simulink model "Control_Arduino"  (R2023b)
settings: Solver=FixedStepDiscrete  StartTime=0.0  StopTime=90  FixedStep=0.01  RelTol=1e-3  EnableMultiTasking=on
undefined symbols (not defined in the file): L, R
libraries: simulink x36, arduinolib x17, canmsglib x4, arduinowifilib x2
settings Model: ExtModeTrigDuration=2  Creator=pablo  LastModifiedBy=pablo
settings SolverCC: AutoInsertRateTranBlk=on
settings OptimizationCC: EnhancedBackFolding=on  PassReuseOutputArgsAs=Individual arguments  ZeroExternalMemoryAtStartup=off  ZeroInternalMemoryAtStartup=off  MaxStackSize=64  OptimizeBlockOrder=speed  DifferentSizesBufferReuse=on  OptimizationCustomize=off  EfficientTunableParamExpr=on
settings DebuggingCC: ReadBeforeWriteMsg=DisableAll  WriteAfterWriteMsg=DisableAll  WriteAfterReadMsg=DisableAll  MultiTaskDSMMsg=none  ParameterTunabilityLossMsg=error
settings HardwareCC: ProdBitPerPointer=32  ProdBitPerSizeT=32  ProdBitPerPtrDiffT=32  ProdLargestAtomicInteger=Long  ProdLargestAtomicFloat=Double  ProdWordSize=32  ProdHWDeviceType=ARM Compatible->ARM Cortex
settings ModelReferenceCC: UpdateModelReferenceTargets=IfOutOfDate
settings SFSimCC: SFSimEcho=off  MATLABDynamicMemAlloc=off
settings RTWCC: Description=Embedded Coder  SystemTargetFile=ert.tlc  HardwareBoard=Arduino MKR WiFi 1010  TemplateMakefile=ert_default_tmf  Toolchain=Arduino ARM  BuildConfiguration=Faster Runs
settings CodeAppCC: ForceParamTrailComments=on  IgnoreCustomStorageClasses=off  OperatorAnnotations=on  SimulinkDataObjDesc=on  SFDataObjDesc=on  InsertBlockDesc=on
settings ERTTargetCC: SupportContinuousTime=on  SupportVariableSizeSignals=on  ExtModeTransport=3  ExtModeStaticAlloc=on  ExtModeAutomaticAllocSize=off  ExtModeStaticAllocSize=8192  ExtModeMexFile=ext_xcp  ExtModeIntrfLevel=Level2 - Open

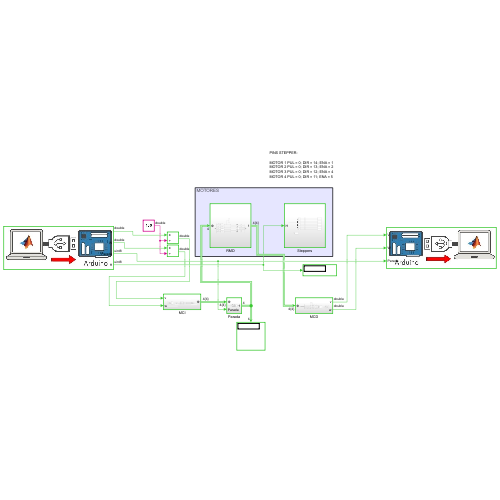
[thumbnail: Simulink's stored preview of the top-level diagram]
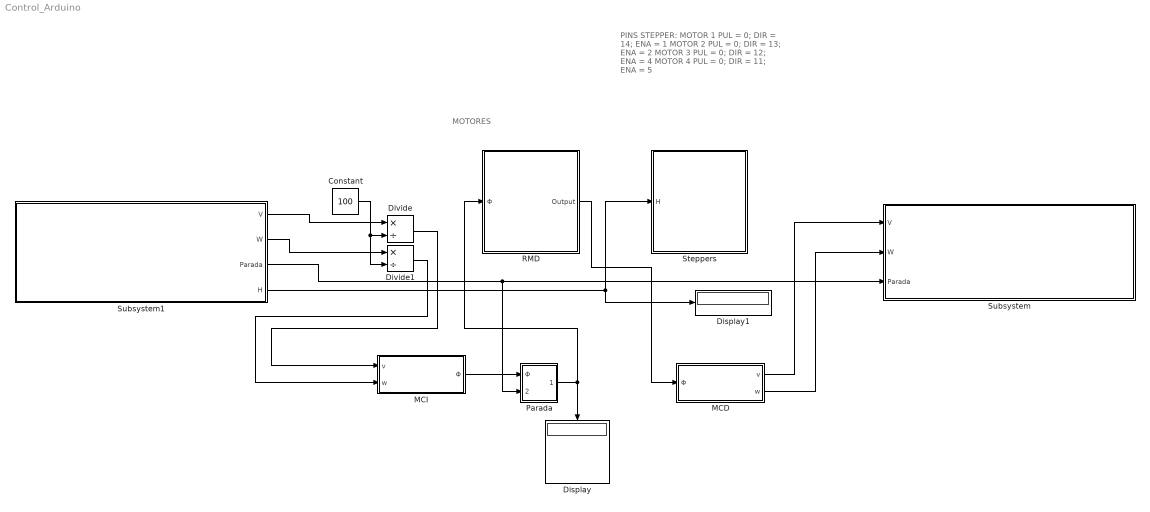
== system Control_Arduino ==
  note: PINS STEPPER:
      |
      | MOTOR 1 PUL = 0; DIR = 14; ENA = 1
      | MOTOR 2 PUL = 0; DIR = 13; ENA = 2
      | MOTOR 3 PUL = 0; DIR = 12; ENA = 4
      | MOTOR 4 PUL = 0; DIR = 11; ENA = 5
  note: MOTORES
  Constant : Constant  Value=100
  Display : Display
  Display1 : Display
      settings: Format=binary (Stored Integer)
  Divide : Product  Inputs=*/
  Divide1 : Product  Inputs=*/
  MCD : Subsystem
  MCI : Subsystem
  Parada : Subsystem
  RMD : Subsystem
  Steppers : Subsystem
  Subsystem : Subsystem
      mask Display: image('am.jpg');
  Subsystem1 : Subsystem
      mask Display: image('ma.jpg');
  wires:
  Subsystem1/1(V) -> Divide/1
  Subsystem1/2(W) -> Divide1/1
  Subsystem1/3(Parada) -> Subsystem/3(Parada), Parada/2(Parada)
  Constant/1 -> Divide1/2, Divide/2
  Divide/1 -> MCI/1(v)
  Divide1/1 -> MCI/2(w)
  MCD/1(v) -> Subsystem/1(V)
  MCD/2(w) -> Subsystem/2(W)
  MCI/1(Φ) -> Parada/1(Φ)
  Parada/1(Out1) -> RMD/1(Φ), Display/1
  RMD/1(Output) -> MCD/1(Φ)
  Subsystem1/4(H) -> Steppers/1(H), Display1/1

== system Control_Arduino/MCD ==
  Φ : Inport
  Bus Selector : BusSelector  OutputSignals=GPS1,GPS2,GPS3,GPS4
  Constant : Constant  Value=2
  Demux : Demux  Outputs=2
  Divide2 : Product  Inputs=*/
  Divide3 : Product  Inputs=*/
  Gain1 : Gain  Gain=[1/2 1/2; -1/L 1/L]  Multiplication=Matrix(K*u) (u vector)
  Gain2 : Gain  Gain=R
  Gain3 : Gain  Gain=R
  Mux : Mux  Inputs=2
  Sum : Sum  Inputs=|++
  Sum1 : Sum  Inputs=|++
  v : Outport
  w : Outport  Port=2
  wires:
  Sum1/1 -> Divide2/1
  Φ/1 -> Bus Selector/1
  Constant/1 -> Divide3/2, Divide2/2
  Sum/1 -> Divide3/1
  Gain2/1 -> Mux/1
  Gain3/1 -> Mux/2
  Mux/1 -> Gain1/1
  Gain1/1 -> Demux/1
  Demux/1 -> v/1
  Demux/2 -> w/1
  Divide2/1 -> Gain2/1
  Divide3/1 -> Gain3/1
  Bus Selector/1 -> Sum1/1  "<GPS1>"
  Bus Selector/2 -> Sum1/2  "<GPS2>"
  Bus Selector/3 -> Sum/1  "<GPS3>"
  Bus Selector/4 -> Sum/2  "<GPS4>"

== system Control_Arduino/MCI ==
  note: velocidad en grados por segundo
  note: L = distancia entre el eje de las ruedas izquierda y derecha
  note: radio de las ruedas
  note: Velocidades angulares:
      | 1. Frente izquierda
      | 2. Trasera izquierda
      | 3. Frente derecha
      | 4. Trasera derecha
  v : Inport
  w : Inport  Port=2
  Bus Creator : BusCreator  Inputs=4
  Demux : Demux  Outputs=2
  Gain : Gain  Gain=[1 -L/2; 1 L/2]  Multiplication=Matrix(K*u) (u vector)
  Gain1 : Gain  Gain=10
  Gain2 : Gain  Gain=1/R
  Gain3 : Gain  Gain=10
  Mux : Mux  Inputs=2
  Rate Limiter : RateLimiter  RisingSlewLimit=9  FallingSlewLimit=-9  SampleTimeMode=inherited
  Rate Limiter1 : RateLimiter  RisingSlewLimit=9  FallingSlewLimit=-9  SampleTimeMode=inherited
  Φ : Outport
  wires:
  Bus Creator/1 -> Φ/1
  Mux/1 -> Gain/1
  v/1 -> Mux/1
  w/1 -> Mux/2
  Demux/1 -> Rate Limiter/1
  Demux/2 -> Rate Limiter1/1
  Gain/1 -> Gain2/1
  Gain2/1 -> Demux/1
  Gain1/1 -> Bus Creator/2, Bus Creator/1
  Rate Limiter1/1 -> Gain3/1
  Rate Limiter/1 -> Gain1/1
  Gain3/1 -> Bus Creator/4, Bus Creator/3

== system Control_Arduino/Parada ==
  Φ : Inport
  Parada : Inport  Port=2
  Bus Creator : BusCreator  Inputs=4
  Constant : Constant  Value=0
  Switch : Switch  Criteria=u2 ~= 0  SaturateOnIntegerOverflow=off  InputSameDT=off
  Out1 : Outport
  wires:
  Switch/1 -> Out1/1
  Φ/1 -> Switch/3
  Parada/1 -> Switch/2
  Bus Creator/1 -> Switch/1
  Constant/1 -> Bus Creator/2, Bus Creator/4, Bus Creator/3, Bus Creator/1

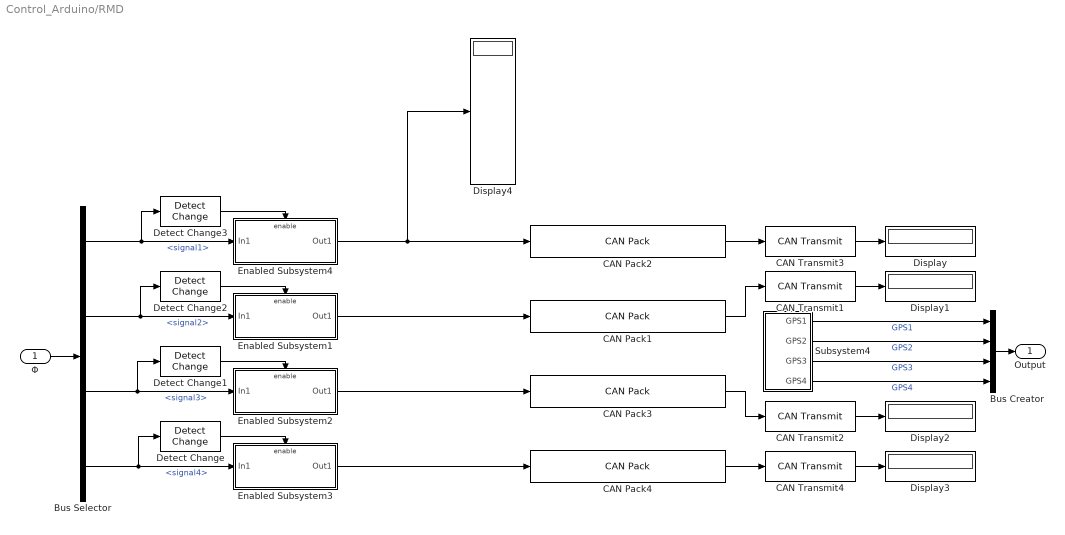
== system Control_Arduino/RMD ==
  Φ : Inport
  Bus Creator : BusCreator  Inputs=4
  Bus Selector : BusSelector  OutputSignals=signal1,signal2,signal3,signal4
  CAN Pack1 : canmsglib/CAN Pack  MsgList=(none)  MsgName=CAN Msg  MsgIDType=Standard (11-bit identifier)  MsgIdentifier=322  MsgLength=8  Remote=off  ApplyMinMax=off  BusOutput=on  SignalInfo={ 'position', '8', '16', 'BE', 'signed', 'Standard', '0', '1', '-95.5', '-95.5', '95.5'; 'velocity', '28', '12', 'BE', 'signed', 'Standard', '0', '1', '-45', '-45', '45'; 'kp', '32', '12', 'BE', 'unsigned', 'Standard', '0', '1', '0', '0', '500'; 'kd', '52', '12', 'BE', 'unsigned', 'Standard', '0', '1', '0', '0', '5'; 'torque', '56', '12', 'BE', 'signed', 'Standard', '0', '1', '-18', '-18', '18' }
      settings: LibrarySourceBlock=embeddedtargetslib/Host Communication/CAN Pack  DataFormat=raw data
  CAN Pack2 : canmsglib/CAN Pack  MsgList=(none)  MsgName=CAN Msg  MsgIDType=Standard (11-bit identifier)  MsgIdentifier=321  MsgLength=8  Remote=off  ApplyMinMax=off  BusOutput=on  SignalInfo={ 'position', '8', '16', 'BE', 'signed', 'Standard', '0', '1', '-95.5', '-95.5', '95.5'; 'velocity', '28', '12', 'BE', 'signed', 'Standard', '0', '1', '-45', '-45', '45'; 'kp', '32', '12', 'BE', 'unsigned', 'Standard', '0', '1', '0', '0', '500'; 'kd', '52', '12', 'BE', 'unsigned', 'Standard', '0', '1', '0', '0', '5'; 'torque', '56', '12', 'BE', 'signed', 'Standard', '0', '1', '-18', '-18', '18' }
      settings: LibrarySourceBlock=embeddedtargetslib/Host Communication/CAN Pack  DataFormat=raw data
  CAN Pack3 : canmsglib/CAN Pack  MsgList=(none)  MsgName=CAN Msg  MsgIDType=Standard (11-bit identifier)  MsgIdentifier=323  MsgLength=8  Remote=off  ApplyMinMax=off  BusOutput=on  SignalInfo={ 'position', '8', '16', 'BE', 'signed', 'Standard', '0', '1', '-95.5', '-95.5', '95.5'; 'velocity', '28', '12', 'BE', 'signed', 'Standard', '0', '1', '-45', '-45', '45'; 'kp', '32', '12', 'BE', 'unsigned', 'Standard', '0', '1', '0', '0', '500'; 'kd', '52', '12', 'BE', 'unsigned', 'Standard', '0', '1', '0', '0', '5'; 'torque', '56', '12', 'BE', 'signed', 'Standard', '0', '1', '-18', '-18', '18' }
      settings: LibrarySourceBlock=embeddedtargetslib/Host Communication/CAN Pack  DataFormat=raw data
  CAN Pack4 : canmsglib/CAN Pack  MsgList=(none)  MsgName=CAN Msg  MsgIDType=Standard (11-bit identifier)  MsgIdentifier=324  MsgLength=8  Remote=off  ApplyMinMax=off  BusOutput=on  SignalInfo={ 'position', '8', '16', 'BE', 'signed', 'Standard', '0', '1', '-95.5', '-95.5', '95.5'; 'velocity', '28', '12', 'BE', 'signed', 'Standard', '0', '1', '-45', '-45', '45'; 'kp', '32', '12', 'BE', 'unsigned', 'Standard', '0', '1', '0', '0', '500'; 'kd', '52', '12', 'BE', 'unsigned', 'Standard', '0', '1', '0', '0', '5'; 'torque', '56', '12', 'BE', 'signed', 'Standard', '0', '1', '-18', '-18', '18' }
      settings: LibrarySourceBlock=embeddedtargetslib/Host Communication/CAN Pack  DataFormat=raw data
  CAN Transmit{1..4} (4 alike) : arduinolib/CAN Transmit  inputDataType=CAN Msg  BlockingMode_=on  BlockTimeout_=1  outputStatus=on  identifierType=Standard (11-bit identifier)  messageId=100  msgLength=8  remoteFrame=off
  Detect Change{,1..3} (4 alike) : simulink/Logic and Bit Operations/Detect Change  vinit=0  OutDataTypeStr=boolean
  Display{,1..4} (5 alike) : Display
      Display settings: Format=binary (Stored Integer)
      Display1 settings: Format=binary (Stored Integer)
      Display2 settings: Format=binary (Stored Integer)
      Display3 settings: Format=binary (Stored Integer)
      Display4 settings: Format=hex (Stored Integer)
  Enabled Subsystem1 : Subsystem  TreatAsAtomicUnit=on
  Enabled Subsystem2 : Subsystem  TreatAsAtomicUnit=on
  Enabled Subsystem3 : Subsystem  TreatAsAtomicUnit=on
  Enabled Subsystem4 : Subsystem  TreatAsAtomicUnit=on
  Subsystem4 : Subsystem
  Output : Outport
  wires:
  Enabled Subsystem4/1(Out1) -> Display4/1, CAN Pack2/1
  Enabled Subsystem1/1(Out1) -> CAN Pack1/1
  Enabled Subsystem2/1(Out1) -> CAN Pack3/1
  Enabled Subsystem3/1(Out1) -> CAN Pack4/1
  CAN Pack2/1 -> CAN Transmit3/1
  CAN Pack4/1 -> CAN Transmit4/1
  CAN Transmit3/1 -> Display/1
  CAN Transmit1/1 -> Display1/1
  CAN Transmit2/1 -> Display2/1
  CAN Transmit4/1 -> Display3/1
  CAN Pack1/1 -> CAN Transmit1/1
  CAN Pack3/1 -> CAN Transmit2/1
  Detect Change/1 -> Enabled Subsystem3/Enable
  Detect Change1/1 -> Enabled Subsystem2/Enable
  Detect Change2/1 -> Enabled Subsystem1/Enable
  Detect Change3/1 -> Enabled Subsystem4/Enable
  Φ/1 -> Bus Selector/1
  Bus Selector/1 -> Enabled Subsystem4/1(In1), Detect Change3/1  "<signal1>"
  Bus Selector/2 -> Detect Change2/1, Enabled Subsystem1/1(In1)  "<signal2>"
  Bus Selector/3 -> Detect Change1/1, Enabled Subsystem2/1(In1)  "<signal3>"
  Bus Selector/4 -> Detect Change/1, Enabled Subsystem3/1(In1)  "<signal4>"
  Subsystem4/1(GPS1) -> Bus Creator/1  "GPS1"
  Subsystem4/2(GPS2) -> Bus Creator/2  "GPS2"
  Subsystem4/3(GPS3) -> Bus Creator/3  "GPS3"
  Subsystem4/4(GPS4) -> Bus Creator/4  "GPS4"
  Bus Creator/1 -> Output/1

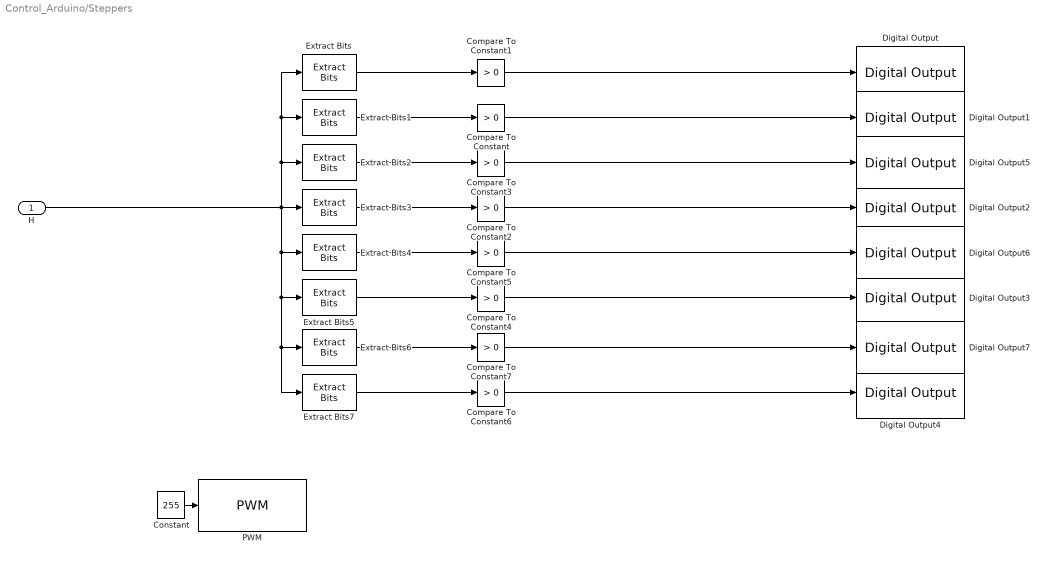
== system Control_Arduino/Steppers ==
  H : Inport
  Compare To Constant{,1..7} (8 alike) : simulink/Logic and Bit Operations/Compare To Constant  relop=>  const=0  OutDataTypeStr=uint8
  Constant : Constant  Value=255
  Digital Output : arduinolib/Digital Output  pinNumber=1  Direction=output  blockPlatform=arduino
  Digital Output1 : arduinolib/Digital Output  pinNumber=14  Direction=output  blockPlatform=arduino
  Digital Output2 : arduinolib/Digital Output  pinNumber=13  Direction=output  blockPlatform=arduino
  Digital Output3 : arduinolib/Digital Output  pinNumber=12  Direction=output  blockPlatform=arduino
  Digital Output4 : arduinolib/Digital Output  pinNumber=11  Direction=output  blockPlatform=arduino
  Digital Output5 : arduinolib/Digital Output  pinNumber=2  Direction=output  blockPlatform=arduino
  Digital Output6 : arduinolib/Digital Output  pinNumber=4  Direction=output  blockPlatform=arduino
  Digital Output7 : arduinolib/Digital Output  pinNumber=5  Direction=output  blockPlatform=arduino
  Extract Bits : simulink/Logic and Bit Operations/Extract Bits  bitsToExtract=Range of bits  numBits=8  bitIdxRange=4  outScalingMode=Preserve fixed-point scaling
  Extract Bits1 : simulink/Logic and Bit Operations/Extract Bits  bitsToExtract=Range of bits  numBits=8  bitIdxRange=0  outScalingMode=Preserve fixed-point scaling
  Extract Bits2 : simulink/Logic and Bit Operations/Extract Bits  bitsToExtract=Range of bits  numBits=8  bitIdxRange=5  outScalingMode=Preserve fixed-point scaling
  Extract Bits3 : simulink/Logic and Bit Operations/Extract Bits  bitsToExtract=Range of bits  numBits=8  bitIdxRange=1  outScalingMode=Preserve fixed-point scaling
  Extract Bits4 : simulink/Logic and Bit Operations/Extract Bits  bitsToExtract=Range of bits  numBits=8  bitIdxRange=6  outScalingMode=Preserve fixed-point scaling
  Extract Bits5 : simulink/Logic and Bit Operations/Extract Bits  bitsToExtract=Range of bits  numBits=8  bitIdxRange=2  outScalingMode=Preserve fixed-point scaling
  Extract Bits6 : simulink/Logic and Bit Operations/Extract Bits  bitsToExtract=Range of bits  numBits=8  bitIdxRange=7  outScalingMode=Preserve fixed-point scaling
  Extract Bits7 : simulink/Logic and Bit Operations/Extract Bits  bitsToExtract=Range of bits  numBits=8  bitIdxRange=3  outScalingMode=Preserve fixed-point scaling
  PWM : arduinolib/PWM  pinNumber=0  frequencyType=Default  desiredFrequency=490.2  achievableFrequency=490.2
  wires:
  Extract Bits5/1 -> Compare To Constant4/1
  Compare To Constant3/1 -> Digital Output5/1
  Compare To Constant5/1 -> Digital Output6/1
  Compare To Constant2/1 -> Digital Output2/1
  Extract Bits7/1 -> Compare To Constant6/1
  Compare To Constant4/1 -> Digital Output3/1
  Compare To Constant7/1 -> Digital Output7/1
  Extract Bits/1 -> Compare To Constant1/1
  Compare To Constant/1 -> Digital Output1/1
  Compare To Constant1/1 -> Digital Output/1
  Extract Bits2/1 -> Compare To Constant3/1
  Extract Bits4/1 -> Compare To Constant5/1
  Compare To Constant6/1 -> Digital Output4/1
  Extract Bits3/1 -> Compare To Constant2/1
  Extract Bits1/1 -> Compare To Constant/1
  Extract Bits6/1 -> Compare To Constant7/1
  H/1 -> Extract Bits3/1, Extract Bits2/1, Extract Bits1/1, Extract Bits/1, Extract Bits4/1, Extract Bits5/1, Extract Bits7/1, Extract Bits6/1
  Constant/1 -> PWM/1

== system Control_Arduino/Subsystem ==
  V : Inport
  W : Inport  Port=2
  Parada : Inport  Port=3
  Data Type Conversion1 : DataTypeConversion  OutDataTypeStr=int16  ConvertRealWorld=Stored Integer (SI)  SaturateOnIntegerOverflow=off  RndMeth=Floor
  Data Type Conversion6 : DataTypeConversion  OutDataTypeStr=int16  ConvertRealWorld=Stored Integer (SI)  SaturateOnIntegerOverflow=off  RndMeth=Floor
  Data Type Conversion7 : DataTypeConversion  OutDataTypeStr=int16  ConvertRealWorld=Stored Integer (SI)  SaturateOnIntegerOverflow=off  RndMeth=Floor
  Display : Display
  Gain : Gain  Gain=100
  Gain5 : Gain  Gain=100
  Mux : Mux  Inputs=3
  WiFi UDP Send : arduinowifilib/WiFi UDP Send  remoteIPOctetString=192.168.137.1  remoteport=8888  localport=9090  remoteipoctet1=192  remoteipoctet2=168  remoteipoctet3=137  remoteipoctet4=1  wifiUDPIndex=0  blockPlatform=ARDUINO  isARMArch=true
  wires:
  Mux/1 -> Display/1, WiFi UDP Send/1
  V/1 -> Gain/1
  W/1 -> Gain5/1
  Data Type Conversion6/1 -> Mux/2
  Data Type Conversion7/1 -> Mux/3
  Gain/1 -> Data Type Conversion1/1
  Gain5/1 -> Data Type Conversion6/1
  Parada/1 -> Data Type Conversion7/1
  Data Type Conversion1/1 -> Mux/1

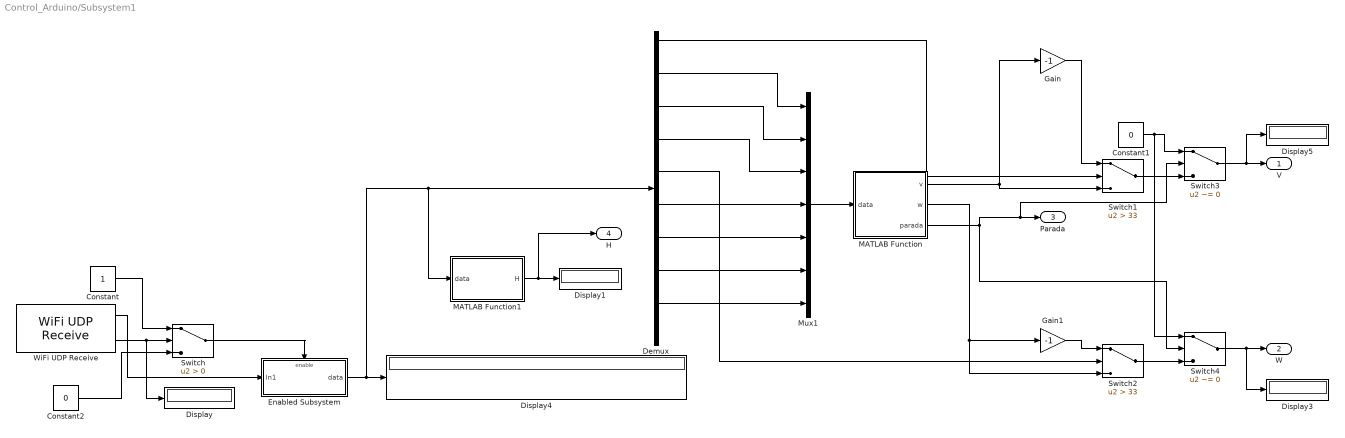
== system Control_Arduino/Subsystem1 ==
  Constant : Constant  OutDataTypeStr=boolean
  Constant1 : Constant  Value=0
  Constant2 : Constant  Value=0  OutDataTypeStr=boolean
  Demux : Demux  Outputs=10
  Display{,1,3..5} (5 alike) : Display
      Display1 settings: Format=binary (Stored Integer)
  Enabled Subsystem : Subsystem  TreatAsAtomicUnit=on
  Gain : Gain  Gain=-1
  Gain1 : Gain  Gain=-1
  MATLAB Function : MATLAB Function  TreatAsAtomicUnit=on
  MATLAB Function1 : MATLAB Function  TreatAsAtomicUnit=on
  Mux1 : Mux  Inputs=7
  Switch : Switch  Criteria=u2 > Threshold  SaturateOnIntegerOverflow=off  InputSameDT=off
  Switch1 : Switch  Criteria=u2 > Threshold  Threshold=33  SaturateOnIntegerOverflow=off  InputSameDT=off
  Switch2 : Switch  Criteria=u2 > Threshold  Threshold=33  SaturateOnIntegerOverflow=off  InputSameDT=off
  Switch3 : Switch  Criteria=u2 ~= 0  SaturateOnIntegerOverflow=off  InputSameDT=off
  Switch4 : Switch  Criteria=u2 ~= 0  SaturateOnIntegerOverflow=off  InputSameDT=off
  WiFi UDP Receive : arduinowifilib/WiFi UDP Receive  localport=9090  DataType=uint8  DataLength=10  SampleTime_=0.1  wifiUDPIndex=0  blockPlatform=ARDUINO  isARMArch=true
  V : Outport
  W : Outport  Port=2
  Parada : Outport  Port=3
  H : Outport  Port=4
  wires:
  Enabled Subsystem/1(data) -> Display4/1, Demux/1, MATLAB Function1/1(data)
  Constant/1 -> Switch/1
  WiFi UDP Receive/1 -> Enabled Subsystem/1(In1)
  Demux/1 -> Switch1/2
  Demux/2 -> Mux1/1
  WiFi UDP Receive/2 -> Switch/2, Display/1
  Demux/4 -> Mux1/3
  Demux/3 -> Mux1/2
  Switch/1 -> Enabled Subsystem/Enable
  Demux/6 -> Mux1/4
  Demux/5 -> Switch2/2
  Demux/8 -> Mux1/6
  Demux/7 -> Mux1/5
  Demux/9 -> Mux1/7
  Mux1/1 -> MATLAB Function/1(data)
  MATLAB Function/1(v) -> Switch1/3, Gain/1
  MATLAB Function/2(w) -> Switch2/3, Gain1/1
  MATLAB Function/3(parada) -> Switch4/2, Switch3/2, Parada/1
  Gain/1 -> Switch1/1
  Gain1/1 -> Switch2/1
  Constant1/1 -> Switch4/1, Switch3/1
  Switch2/1 -> Switch4/3
  Switch1/1 -> Switch3/3
  Switch4/1 -> W/1, Display3/1
  Switch3/1 -> V/1, Display5/1
  MATLAB Function1/1(H) -> H/1, Display1/1
  Constant2/1 -> Switch/3

== system Control_Arduino/RMD/Enabled Subsystem1 ==
  In1 : Inport
  Enable : EnablePort
  Gain : Gain  Gain=100
  Subsystem : Subsystem
  Out1 : Outport
  wires:
  In1/1 -> Gain/1
  Subsystem/1(Out1) -> Out1/1
  Gain/1 -> Subsystem/1(In1)

== system Control_Arduino/RMD/Enabled Subsystem2 ==
  In1 : Inport
  Enable : EnablePort
  Gain : Gain  Gain=100
  Subsystem : Subsystem
  Out1 : Outport
  wires:
  In1/1 -> Gain/1
  Subsystem/1(Out1) -> Out1/1
  Gain/1 -> Subsystem/1(In1)

== system Control_Arduino/RMD/Enabled Subsystem3 ==
  In1 : Inport
  Enable : EnablePort
  Gain : Gain  Gain=100
  Subsystem : Subsystem
  Out1 : Outport
  wires:
  In1/1 -> Gain/1
  Subsystem/1(Out1) -> Out1/1
  Gain/1 -> Subsystem/1(In1)

== system Control_Arduino/RMD/Enabled Subsystem4 ==
  In1 : Inport
  Enable : EnablePort
  Gain : Gain  Gain=100
  Subsystem : Subsystem
  Out1 : Outport
  wires:
  In1/1 -> Gain/1
  Subsystem/1(Out1) -> Out1/1
  Gain/1 -> Subsystem/1(In1)

== system Control_Arduino/RMD/Subsystem4 ==
  CAN Receive : arduinolib/CAN Receive  outputDataType=Raw data  identifierType=Standard (11-bit identifier)  messageId=577  msgLength=8  SampleTime=0.1  outputError=off  outputRemote=off
  CAN Receive1 : arduinolib/CAN Receive  outputDataType=Raw data  identifierType=Standard (11-bit identifier)  messageId=578  msgLength=8  SampleTime=0.1  outputError=off  outputRemote=off
  CAN Receive2 : arduinolib/CAN Receive  outputDataType=Raw data  identifierType=Standard (11-bit identifier)  messageId=579  msgLength=8  SampleTime=0.1  outputError=off  outputRemote=off
  CAN Receive3 : arduinolib/CAN Receive  outputDataType=Raw data  identifierType=Standard (11-bit identifier)  messageId=580  msgLength=8  SampleTime=0.1  outputError=off  outputRemote=off
  Subsystem : Subsystem
  Subsystem1 : Subsystem
  Subsystem2 : Subsystem
  Subsystem3 : Subsystem
  GPS1 : Outport
  GPS2 : Outport  Port=2
  GPS3 : Outport  Port=3
  GPS4 : Outport  Port=4
  wires:
  CAN Receive1/1 -> Subsystem2/1(In1)
  CAN Receive3/1 -> Subsystem/1(In1)
  CAN Receive2/1 -> Subsystem3/1(In1)
  CAN Receive/1 -> Subsystem1/1(In1)
  CAN Receive1/2 -> Subsystem2/Enable
  CAN Receive3/2 -> Subsystem/Enable
  CAN Receive2/2 -> Subsystem3/Enable
  CAN Receive/2 -> Subsystem1/Enable
  Subsystem1/1(GPS1) -> GPS1/1
  Subsystem3/1(GPS3) -> GPS3/1
  Subsystem/1(GPS4) -> GPS4/1
  Subsystem2/1(GPS2) -> GPS2/1

== system Control_Arduino/Subsystem1/Enabled Subsystem ==
  In1 : Inport
  Enable : EnablePort
  data : Outport
  wires:
  In1/1 -> data/1

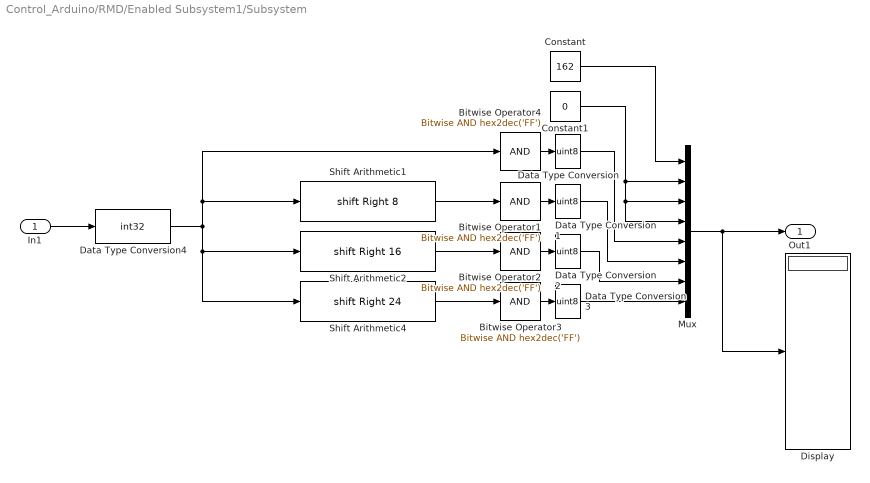
== system Control_Arduino/RMD/Enabled Subsystem1/Subsystem ==
  In1 : Inport
  Bitwise Operator{1..4} (4 alike) : simulink/Logic and Bit Operations/Bitwise Operator  logicop=AND  UseBitMask=on  BitMask=hex2dec('FF')  BitMaskRealWorld=Stored Integer
  Constant : Constant  Value=162  OutDataTypeStr=uint8
  Constant1 : Constant  Value=0  OutDataTypeStr=uint8
  Data Type Conversion{,1..3} (4 alike) : DataTypeConversion  OutDataTypeStr=uint8  ConvertRealWorld=Stored Integer (SI)  SaturateOnIntegerOverflow=off  RndMeth=Floor
  Data Type Conversion4 : DataTypeConversion  OutDataTypeStr=int32  SaturateOnIntegerOverflow=off  RndMeth=Floor
  Display : Display
  Mux : Mux  Inputs=8
  Shift Arithmetic1 : ArithShift  BitShiftNumber=8  BinPtShiftNumber=32  BitShiftDirection=Right
  Shift Arithmetic2 : ArithShift  BitShiftNumber=16  BinPtShiftNumber=32  BitShiftDirection=Right
  Shift Arithmetic4 : ArithShift  BitShiftNumber=24  BinPtShiftNumber=32  BitShiftDirection=Right
  Out1 : Outport
  wires:
  Bitwise Operator4/1 -> Data Type Conversion/1
  Shift Arithmetic1/1 -> Bitwise Operator1/1
  Bitwise Operator1/1 -> Data Type Conversion1/1
  Shift Arithmetic2/1 -> Bitwise Operator2/1
  Bitwise Operator2/1 -> Data Type Conversion2/1
  Shift Arithmetic4/1 -> Bitwise Operator3/1
  Bitwise Operator3/1 -> Data Type Conversion3/1
  Data Type Conversion4/1 -> Shift Arithmetic2/1, Shift Arithmetic4/1, Shift Arithmetic1/1, Bitwise Operator4/1
  In1/1 -> Data Type Conversion4/1
  Mux/1 -> Display/1, Out1/1
  Constant/1 -> Mux/1
  Constant1/1 -> Mux/4, Mux/3, Mux/2
  Data Type Conversion/1 -> Mux/5
  Data Type Conversion1/1 -> Mux/6
  Data Type Conversion2/1 -> Mux/7
  Data Type Conversion3/1 -> Mux/8

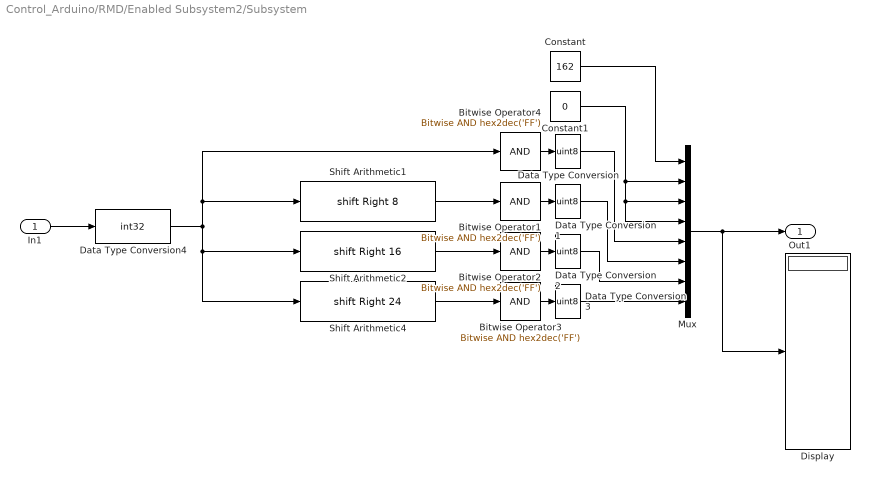
== system Control_Arduino/RMD/Enabled Subsystem2/Subsystem ==
  In1 : Inport
  Bitwise Operator{1..4} (4 alike) : simulink/Logic and Bit Operations/Bitwise Operator  logicop=AND  UseBitMask=on  BitMask=hex2dec('FF')  BitMaskRealWorld=Stored Integer
  Constant : Constant  Value=162  OutDataTypeStr=uint8
  Constant1 : Constant  Value=0  OutDataTypeStr=uint8
  Data Type Conversion{,1..3} (4 alike) : DataTypeConversion  OutDataTypeStr=uint8  ConvertRealWorld=Stored Integer (SI)  SaturateOnIntegerOverflow=off  RndMeth=Floor
  Data Type Conversion4 : DataTypeConversion  OutDataTypeStr=int32  SaturateOnIntegerOverflow=off  RndMeth=Floor
  Display : Display
  Mux : Mux  Inputs=8
  Shift Arithmetic1 : ArithShift  BitShiftNumber=8  BinPtShiftNumber=32  BitShiftDirection=Right
  Shift Arithmetic2 : ArithShift  BitShiftNumber=16  BinPtShiftNumber=32  BitShiftDirection=Right
  Shift Arithmetic4 : ArithShift  BitShiftNumber=24  BinPtShiftNumber=32  BitShiftDirection=Right
  Out1 : Outport
  wires:
  Bitwise Operator4/1 -> Data Type Conversion/1
  Shift Arithmetic1/1 -> Bitwise Operator1/1
  Bitwise Operator1/1 -> Data Type Conversion1/1
  Shift Arithmetic2/1 -> Bitwise Operator2/1
  Bitwise Operator2/1 -> Data Type Conversion2/1
  Shift Arithmetic4/1 -> Bitwise Operator3/1
  Bitwise Operator3/1 -> Data Type Conversion3/1
  Data Type Conversion4/1 -> Shift Arithmetic2/1, Shift Arithmetic4/1, Shift Arithmetic1/1, Bitwise Operator4/1
  In1/1 -> Data Type Conversion4/1
  Mux/1 -> Display/1, Out1/1
  Constant/1 -> Mux/1
  Constant1/1 -> Mux/4, Mux/3, Mux/2
  Data Type Conversion/1 -> Mux/5
  Data Type Conversion1/1 -> Mux/6
  Data Type Conversion2/1 -> Mux/7
  Data Type Conversion3/1 -> Mux/8

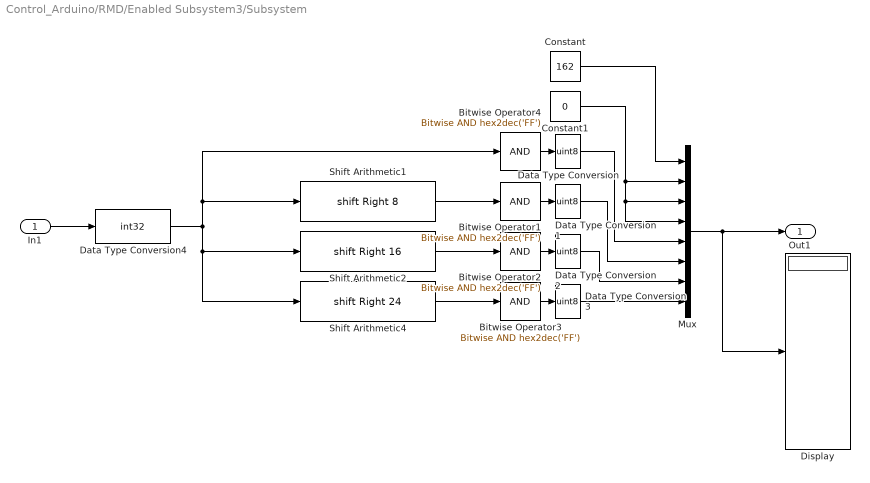
== system Control_Arduino/RMD/Enabled Subsystem3/Subsystem ==
  In1 : Inport
  Bitwise Operator{1..4} (4 alike) : simulink/Logic and Bit Operations/Bitwise Operator  logicop=AND  UseBitMask=on  BitMask=hex2dec('FF')  BitMaskRealWorld=Stored Integer
  Constant : Constant  Value=162  OutDataTypeStr=uint8
  Constant1 : Constant  Value=0  OutDataTypeStr=uint8
  Data Type Conversion{,1..3} (4 alike) : DataTypeConversion  OutDataTypeStr=uint8  ConvertRealWorld=Stored Integer (SI)  SaturateOnIntegerOverflow=off  RndMeth=Floor
  Data Type Conversion4 : DataTypeConversion  OutDataTypeStr=int32  SaturateOnIntegerOverflow=off  RndMeth=Floor
  Display : Display
  Mux : Mux  Inputs=8
  Shift Arithmetic1 : ArithShift  BitShiftNumber=8  BinPtShiftNumber=32  BitShiftDirection=Right
  Shift Arithmetic2 : ArithShift  BitShiftNumber=16  BinPtShiftNumber=32  BitShiftDirection=Right
  Shift Arithmetic4 : ArithShift  BitShiftNumber=24  BinPtShiftNumber=32  BitShiftDirection=Right
  Out1 : Outport
  wires:
  Bitwise Operator4/1 -> Data Type Conversion/1
  Shift Arithmetic1/1 -> Bitwise Operator1/1
  Bitwise Operator1/1 -> Data Type Conversion1/1
  Shift Arithmetic2/1 -> Bitwise Operator2/1
  Bitwise Operator2/1 -> Data Type Conversion2/1
  Shift Arithmetic4/1 -> Bitwise Operator3/1
  Bitwise Operator3/1 -> Data Type Conversion3/1
  Data Type Conversion4/1 -> Shift Arithmetic2/1, Shift Arithmetic4/1, Shift Arithmetic1/1, Bitwise Operator4/1
  In1/1 -> Data Type Conversion4/1
  Mux/1 -> Display/1, Out1/1
  Constant/1 -> Mux/1
  Constant1/1 -> Mux/4, Mux/3, Mux/2
  Data Type Conversion/1 -> Mux/5
  Data Type Conversion1/1 -> Mux/6
  Data Type Conversion2/1 -> Mux/7
  Data Type Conversion3/1 -> Mux/8

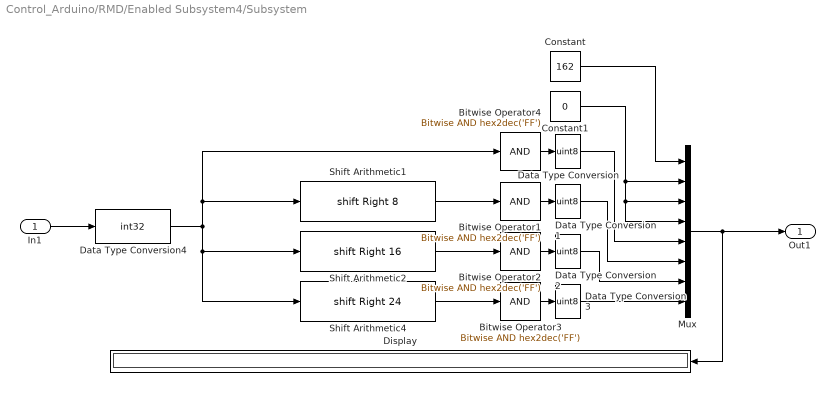
== system Control_Arduino/RMD/Enabled Subsystem4/Subsystem ==
  In1 : Inport
  Bitwise Operator{1..4} (4 alike) : simulink/Logic and Bit Operations/Bitwise Operator  logicop=AND  UseBitMask=on  BitMask=hex2dec('FF')  BitMaskRealWorld=Stored Integer
  Constant : Constant  Value=162  OutDataTypeStr=uint8
  Constant1 : Constant  Value=0  OutDataTypeStr=uint8
  Data Type Conversion{,1..3} (4 alike) : DataTypeConversion  OutDataTypeStr=uint8  ConvertRealWorld=Stored Integer (SI)  SaturateOnIntegerOverflow=off  RndMeth=Floor
  Data Type Conversion4 : DataTypeConversion  OutDataTypeStr=int32  SaturateOnIntegerOverflow=off  RndMeth=Floor
  Display : Display
  Mux : Mux  Inputs=8
  Shift Arithmetic1 : ArithShift  BitShiftNumber=8  BinPtShiftNumber=32  BitShiftDirection=Right
  Shift Arithmetic2 : ArithShift  BitShiftNumber=16  BinPtShiftNumber=32  BitShiftDirection=Right
  Shift Arithmetic4 : ArithShift  BitShiftNumber=24  BinPtShiftNumber=32  BitShiftDirection=Right
  Out1 : Outport
  wires:
  Bitwise Operator4/1 -> Data Type Conversion/1
  Shift Arithmetic1/1 -> Bitwise Operator1/1
  Bitwise Operator1/1 -> Data Type Conversion1/1
  Shift Arithmetic2/1 -> Bitwise Operator2/1
  Bitwise Operator2/1 -> Data Type Conversion2/1
  Shift Arithmetic4/1 -> Bitwise Operator3/1
  Bitwise Operator3/1 -> Data Type Conversion3/1
  Data Type Conversion4/1 -> Shift Arithmetic2/1, Shift Arithmetic4/1, Shift Arithmetic1/1, Bitwise Operator4/1
  In1/1 -> Data Type Conversion4/1
  Mux/1 -> Display/1, Out1/1
  Constant/1 -> Mux/1
  Constant1/1 -> Mux/4, Mux/3, Mux/2
  Data Type Conversion/1 -> Mux/5
  Data Type Conversion1/1 -> Mux/6
  Data Type Conversion2/1 -> Mux/7
  Data Type Conversion3/1 -> Mux/8

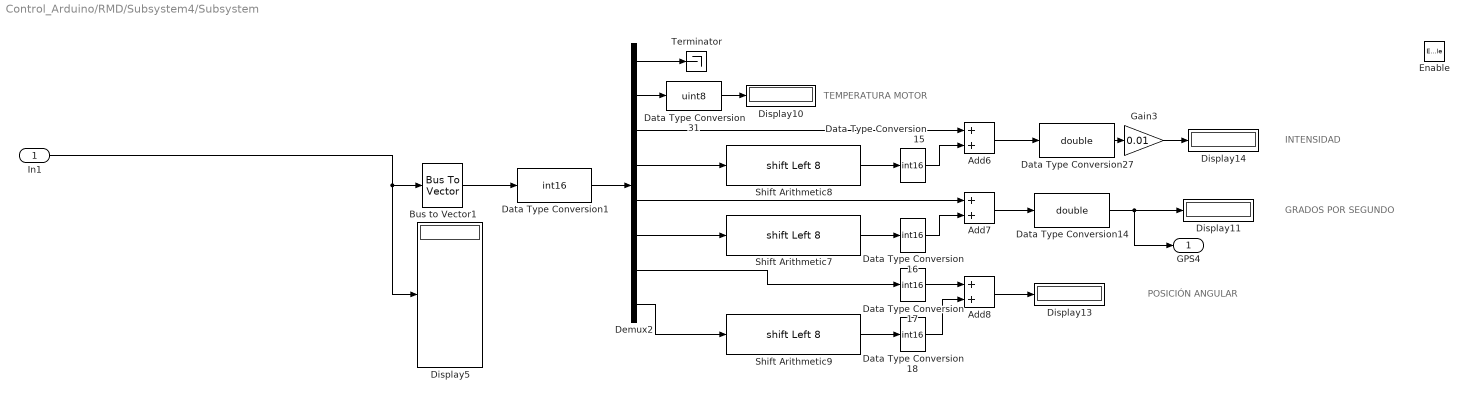
== system Control_Arduino/RMD/Subsystem4/Subsystem ==
  note: TEMPERATURA MOTOR
  note: INTENSIDAD
  note: GRADOS POR SEGUNDO
  note: POSICIÓN ANGULAR
  In1 : Inport
  Enable : EnablePort
  Add6 : Sum
  Add7 : Sum
  Add8 : Sum
  Bus to Vector1 : BusToVector
  Data Type Conversion{1,15..18} (5 alike) : DataTypeConversion  OutDataTypeStr=int16  ConvertRealWorld=Stored Integer (SI)  SaturateOnIntegerOverflow=off  RndMeth=Floor
  Data Type Conversion14 : DataTypeConversion  OutDataTypeStr=double  SaturateOnIntegerOverflow=off  RndMeth=Floor
  Data Type Conversion27 : DataTypeConversion  OutDataTypeStr=double  SaturateOnIntegerOverflow=off  RndMeth=Floor
  Data Type Conversion31 : DataTypeConversion  OutDataTypeStr=uint8  ConvertRealWorld=Stored Integer (SI)  SaturateOnIntegerOverflow=off  RndMeth=Floor
  Demux2 : Demux  Outputs=8
  Display{5,10..11,13..14} (5 alike) : Display
      Display11 settings: Format=decimal (Stored Integer)
      Display13 settings: Format=decimal (Stored Integer)
      Display14 settings: Format=decimal (Stored Integer)
      Display5 settings: Format=hex (Stored Integer)
  Gain3 : Gain  Gain=0.01
  Shift Arithmetic7 : ArithShift  BitShiftNumber=8  BinPtShiftNumber=16  BitShiftDirection=Left
  Shift Arithmetic8 : ArithShift  BitShiftNumber=8  BinPtShiftNumber=16  BitShiftDirection=Left
  Shift Arithmetic9 : ArithShift  BitShiftNumber=8  BinPtShiftNumber=16  BitShiftDirection=Left
  Terminator : Terminator
  GPS4 : Outport
  wires:
  In1/1 -> Display5/1, Bus to Vector1/1
  Data Type Conversion1/1 -> Demux2/1
  Shift Arithmetic9/1 -> Data Type Conversion18/1
  Demux2/1 -> Terminator/1
  Demux2/2 -> Data Type Conversion31/1
  Data Type Conversion14/1 -> GPS4/1, Display11/1
  Demux2/4 -> Shift Arithmetic8/1
  Demux2/8 -> Shift Arithmetic9/1
  Demux2/7 -> Data Type Conversion17/1
  Shift Arithmetic8/1 -> Data Type Conversion15/1
  Demux2/5 -> Add7/1
  Shift Arithmetic7/1 -> Data Type Conversion16/1
  Demux2/3 -> Add6/1
  Demux2/6 -> Shift Arithmetic7/1
  Data Type Conversion16/1 -> Add7/2
  Data Type Conversion17/1 -> Add8/1
  Add8/1 -> Display13/1
  Data Type Conversion27/1 -> Gain3/1
  Add7/1 -> Data Type Conversion14/1
  Gain3/1 -> Display14/1
  Data Type Conversion15/1 -> Add6/2
  Data Type Conversion18/1 -> Add8/2
  Data Type Conversion31/1 -> Display10/1
  Add6/1 -> Data Type Conversion27/1
  Bus to Vector1/1 -> Data Type Conversion1/1

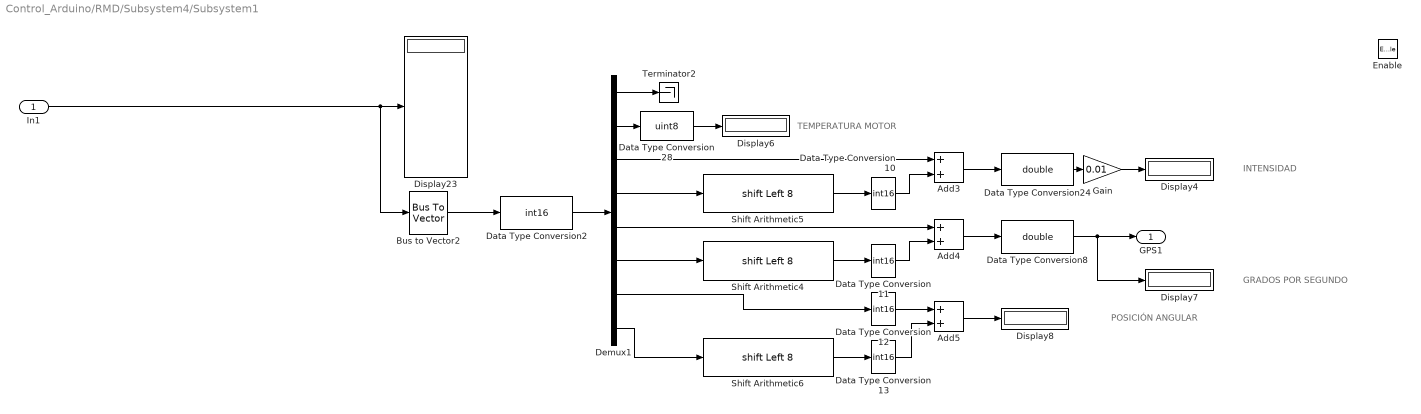
== system Control_Arduino/RMD/Subsystem4/Subsystem1 ==
  note: GRADOS POR SEGUNDO
  note: INTENSIDAD
  note: TEMPERATURA MOTOR
  note: POSICIÓN ANGULAR
  In1 : Inport
  Enable : EnablePort
  Add3 : Sum
  Add4 : Sum
  Add5 : Sum
  Bus to Vector2 : BusToVector
  Data Type Conversion{2,10..13} (5 alike) : DataTypeConversion  OutDataTypeStr=int16  ConvertRealWorld=Stored Integer (SI)  SaturateOnIntegerOverflow=off  RndMeth=Floor
  Data Type Conversion24 : DataTypeConversion  OutDataTypeStr=double  SaturateOnIntegerOverflow=off  RndMeth=Floor
  Data Type Conversion28 : DataTypeConversion  OutDataTypeStr=uint8  ConvertRealWorld=Stored Integer (SI)  SaturateOnIntegerOverflow=off  RndMeth=Floor
  Data Type Conversion8 : DataTypeConversion  OutDataTypeStr=double  SaturateOnIntegerOverflow=off  RndMeth=Floor
  Demux1 : Demux  Outputs=8
  Display{4,6..8,23} (5 alike) : Display
      Display23 settings: Format=hex (Stored Integer)
      Display4 settings: Format=decimal (Stored Integer)
      Display7 settings: Format=decimal (Stored Integer)
      Display8 settings: Format=decimal (Stored Integer)
  Gain : Gain  Gain=0.01
  Shift Arithmetic4 : ArithShift  BitShiftNumber=8  BinPtShiftNumber=16  BitShiftDirection=Left
  Shift Arithmetic5 : ArithShift  BitShiftNumber=8  BinPtShiftNumber=16  BitShiftDirection=Left
  Shift Arithmetic6 : ArithShift  BitShiftNumber=8  BinPtShiftNumber=16  BitShiftDirection=Left
  Terminator2 : Terminator
  GPS1 : Outport
  wires:
  Data Type Conversion2/1 -> Demux1/1
  Demux1/6 -> Shift Arithmetic4/1
  Add4/1 -> Data Type Conversion8/1
  In1/1 -> Display23/1, Bus to Vector2/1
  Demux1/7 -> Data Type Conversion12/1
  Demux1/4 -> Shift Arithmetic5/1
  Demux1/3 -> Add3/1
  Demux1/8 -> Shift Arithmetic6/1
  Bus to Vector2/1 -> Data Type Conversion2/1
  Data Type Conversion13/1 -> Add5/2
  Demux1/2 -> Data Type Conversion28/1
  Shift Arithmetic4/1 -> Data Type Conversion11/1
  Shift Arithmetic6/1 -> Data Type Conversion13/1
  Demux1/5 -> Add4/1
  Data Type Conversion12/1 -> Add5/1
  Add3/1 -> Data Type Conversion24/1
  Data Type Conversion10/1 -> Add3/2
  Add5/1 -> Display8/1
  Data Type Conversion8/1 -> GPS1/1, Display7/1
  Shift Arithmetic5/1 -> Data Type Conversion10/1
  Gain/1 -> Display4/1
  Data Type Conversion11/1 -> Add4/2
  Data Type Conversion28/1 -> Display6/1
  Data Type Conversion24/1 -> Gain/1
  Demux1/1 -> Terminator2/1

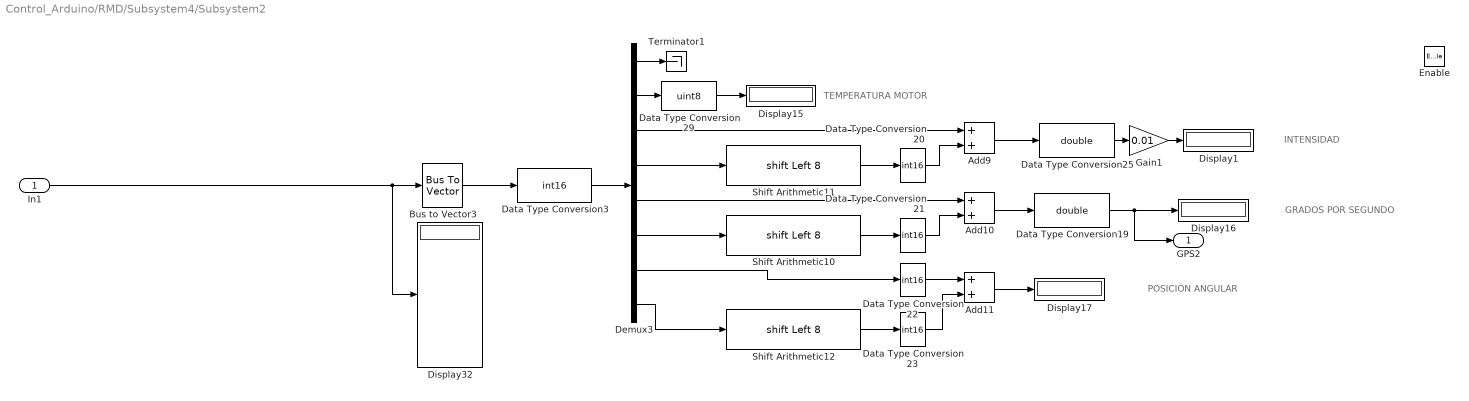
== system Control_Arduino/RMD/Subsystem4/Subsystem2 ==
  note: TEMPERATURA MOTOR
  note: INTENSIDAD
  note: GRADOS POR SEGUNDO
  note: POSICIÓN ANGULAR
  In1 : Inport
  Enable : EnablePort
  Add10 : Sum
  Add11 : Sum
  Add9 : Sum
  Bus to Vector3 : BusToVector
  Data Type Conversion19 : DataTypeConversion  OutDataTypeStr=double  SaturateOnIntegerOverflow=off  RndMeth=Floor
  Data Type Conversion{3,20..23} (5 alike) : DataTypeConversion  OutDataTypeStr=int16  ConvertRealWorld=Stored Integer (SI)  SaturateOnIntegerOverflow=off  RndMeth=Floor
  Data Type Conversion25 : DataTypeConversion  OutDataTypeStr=double  SaturateOnIntegerOverflow=off  RndMeth=Floor
  Data Type Conversion29 : DataTypeConversion  OutDataTypeStr=uint8  ConvertRealWorld=Stored Integer (SI)  SaturateOnIntegerOverflow=off  RndMeth=Floor
  Demux3 : Demux  Outputs=8
  Display{1,15..17,32} (5 alike) : Display
      Display1 settings: Format=decimal (Stored Integer)
      Display16 settings: Format=decimal (Stored Integer)
      Display17 settings: Format=decimal (Stored Integer)
      Display32 settings: Format=hex (Stored Integer)
  Gain1 : Gain  Gain=0.01
  Shift Arithmetic10 : ArithShift  BitShiftNumber=8  BinPtShiftNumber=16  BitShiftDirection=Left
  Shift Arithmetic11 : ArithShift  BitShiftNumber=8  BinPtShiftNumber=16  BitShiftDirection=Left
  Shift Arithmetic12 : ArithShift  BitShiftNumber=8  BinPtShiftNumber=16  BitShiftDirection=Left
  Terminator1 : Terminator
  GPS2 : Outport
  wires:
  In1/1 -> Display32/1, Bus to Vector3/1
  Data Type Conversion3/1 -> Demux3/1
  Demux3/3 -> Add9/1
  Demux3/4 -> Shift Arithmetic11/1
  Bus to Vector3/1 -> Data Type Conversion3/1
  Data Type Conversion20/1 -> Add9/2
  Data Type Conversion19/1 -> GPS2/1, Display16/1
  Demux3/2 -> Data Type Conversion29/1
  Shift Arithmetic12/1 -> Data Type Conversion23/1
  Shift Arithmetic10/1 -> Data Type Conversion21/1
  Data Type Conversion21/1 -> Add10/2
  Demux3/6 -> Shift Arithmetic10/1
  Demux3/8 -> Shift Arithmetic12/1
  Shift Arithmetic11/1 -> Data Type Conversion20/1
  Data Type Conversion22/1 -> Add11/1
  Demux3/1 -> Terminator1/1
  Add10/1 -> Data Type Conversion19/1
  Add11/1 -> Display17/1
  Data Type Conversion23/1 -> Add11/2
  Demux3/5 -> Add10/1
  Add9/1 -> Data Type Conversion25/1
  Data Type Conversion25/1 -> Gain1/1
  Demux3/7 -> Data Type Conversion22/1
  Gain1/1 -> Display1/1
  Data Type Conversion29/1 -> Display15/1

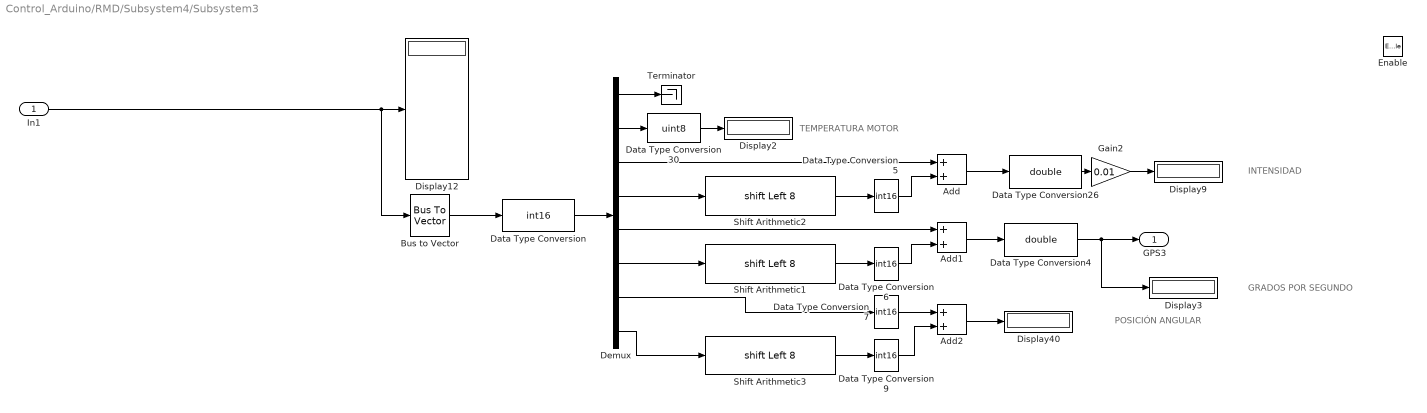
== system Control_Arduino/RMD/Subsystem4/Subsystem3 ==
  note: POSICIÓN ANGULAR
  note: TEMPERATURA MOTOR
  note: INTENSIDAD
  note: GRADOS POR SEGUNDO
  In1 : Inport
  Enable : EnablePort
  Add : Sum
  Add1 : Sum
  Add2 : Sum
  Bus to Vector : BusToVector
  Data Type Conversion{,5..7,9} (5 alike) : DataTypeConversion  OutDataTypeStr=int16  ConvertRealWorld=Stored Integer (SI)  SaturateOnIntegerOverflow=off  RndMeth=Floor
  Data Type Conversion26 : DataTypeConversion  OutDataTypeStr=double  SaturateOnIntegerOverflow=off  RndMeth=Floor
  Data Type Conversion30 : DataTypeConversion  OutDataTypeStr=uint8  ConvertRealWorld=Stored Integer (SI)  SaturateOnIntegerOverflow=off  RndMeth=Floor
  Data Type Conversion4 : DataTypeConversion  OutDataTypeStr=double  SaturateOnIntegerOverflow=off  RndMeth=Floor
  Demux : Demux  Outputs=8
  Display{2..3,9,12,40} (5 alike) : Display
      Display12 settings: Format=hex (Stored Integer)
      Display3 settings: Format=decimal (Stored Integer)
      Display40 settings: Format=decimal (Stored Integer)
      Display9 settings: Format=decimal (Stored Integer)
  Gain2 : Gain  Gain=0.01
  Shift Arithmetic1 : ArithShift  BitShiftNumber=8  BinPtShiftNumber=16  BitShiftDirection=Left
  Shift Arithmetic2 : ArithShift  BitShiftNumber=8  BinPtShiftNumber=16  BitShiftDirection=Left
  Shift Arithmetic3 : ArithShift  BitShiftNumber=8  BinPtShiftNumber=16  BitShiftDirection=Left
  Terminator : Terminator
  GPS3 : Outport
  wires:
  In1/1 -> Display12/1, Bus to Vector/1
  Data Type Conversion/1 -> Demux/1
  Add2/1 -> Display40/1
  Data Type Conversion9/1 -> Add2/2
  Demux/2 -> Data Type Conversion30/1
  Gain2/1 -> Display9/1
  Bus to Vector/1 -> Data Type Conversion/1
  Demux/6 -> Shift Arithmetic1/1
  Demux/1 -> Terminator/1
  Demux/3 -> Add/1
  Demux/4 -> Shift Arithmetic2/1
  Data Type Conversion4/1 -> GPS3/1, Display3/1
  Shift Arithmetic1/1 -> Data Type Conversion6/1
  Data Type Conversion5/1 -> Add/2
  Data Type Conversion7/1 -> Add2/1
  Data Type Conversion6/1 -> Add1/2
  Demux/5 -> Add1/1
  Shift Arithmetic3/1 -> Data Type Conversion9/1
  Demux/8 -> Shift Arithmetic3/1
  Add1/1 -> Data Type Conversion4/1
  Data Type Conversion26/1 -> Gain2/1
  Shift Arithmetic2/1 -> Data Type Conversion5/1
  Demux/7 -> Data Type Conversion7/1
  Data Type Conversion30/1 -> Display2/1
  Add/1 -> Data Type Conversion26/1

== matlab function Control_Arduino/Subsystem1/MATLAB Function ==
  data: data input; v output; w output; parada output
function [v,w,parada] = data2vwparada(data)
parada=uint8(0);
v=single(0);
w=single(0);
d1=single(data(1)-48);
d2=single(data(2)-48);
d3=single(data(3)-48);
d4=single(data(4)-48);
d5=single(data(5)-48);
d6=single(data(6)-48);


v=single(d1*16^2+d2*16+d3);
w=single(d4*16^2+d5*16+d6);
parada=data(7)-48;

== matlab function Control_Arduino/Subsystem1/MATLAB Function1 ==
  data: data input; H output
function H  = extraerH(data)
H=data(10);
end
